simulink model "TD1_2"  (R2022b)
settings: Solver=VariableStepAuto  StartTime=0.0  StopTime=10.0  RelTol=1e-3
values from neighbouring files (symbols this model uses):
  A = [0 1; 1 2]    [temp.m]
  B = [0 ; 1]    [temp.m]
  C = [1 0]    [temp.m]
undefined symbols (not defined in the file or in its folder): h, K, Ki
settings Model: Creator=simon.dumesny  LastModifiedBy=simon.dumesny

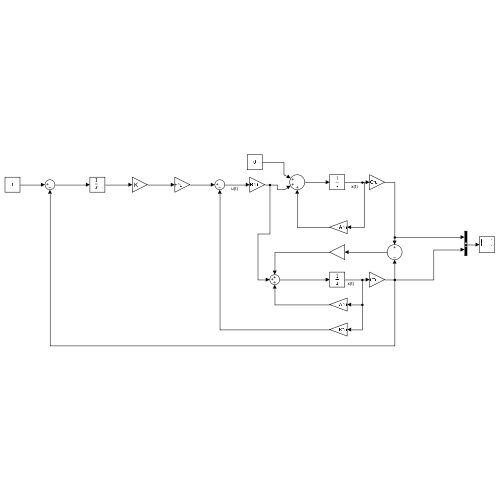
[thumbnail: Simulink's stored preview of the top-level diagram]
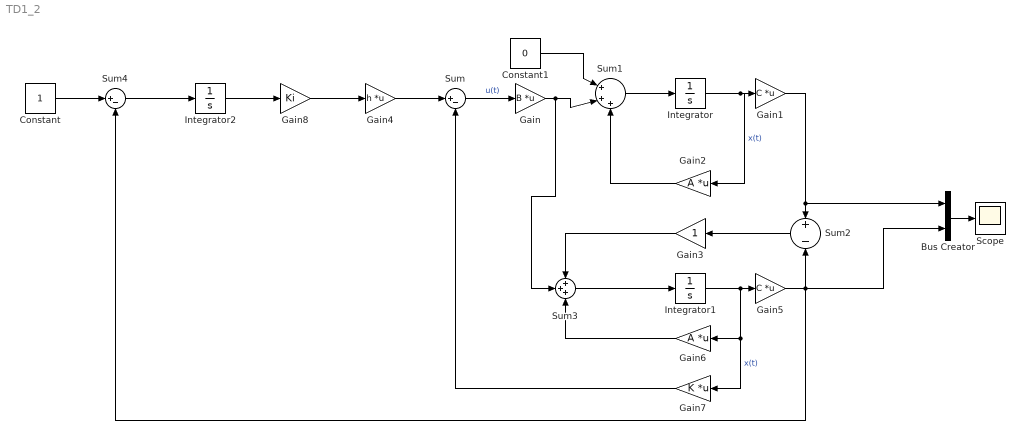
== system TD1_2 ==
  Bus Creator : BusCreator  Inputs=2
  Constant : Constant
  Constant1 : Constant  Value=0
  Gain : Gain  Gain=B  Multiplication=Matrix(K*u)
  Gain1 : Gain  Gain=C  Multiplication=Matrix(K*u)
  Gain2 : Gain  Gain=A  Multiplication=Matrix(K*u)
  Gain3 : Gain
  Gain4 : Gain  Gain=h  Multiplication=Matrix(K*u)
  Gain5 : Gain  Gain=C  Multiplication=Matrix(K*u)
  Gain6 : Gain  Gain=A  Multiplication=Matrix(K*u)
  Gain7 : Gain  Gain=K  Multiplication=Matrix(K*u)
  Gain8 : Gain  Gain=Ki
  Integrator : Integrator
  Integrator1 : Integrator
  Integrator2 : Integrator
  Scope : Scope
  Sum : Sum  Inputs=|+-
  Sum1 : Sum  Inputs=|+++
  Sum2 : Sum  Inputs=+-
  Sum3 : Sum  Inputs=+++
  Sum4 : Sum  Inputs=|+-
  wires:
  Sum/1 -> Gain/1  "u(t)"
  Gain/1 -> Sum3/2, Sum1/2
  Sum1/1 -> Integrator/1
  Constant1/1 -> Sum1/1
  Integrator/1 -> Gain2/1, Gain1/1  "x(t)"
  Gain2/1 -> Sum1/3
  Gain8/1 -> Gain4/1
  Gain4/1 -> Sum/1
  Gain1/1 -> Sum2/1, Bus Creator/1
  Bus Creator/1 -> Scope/1
  Sum2/1 -> Gain3/1
  Gain3/1 -> Sum3/1
  Sum3/1 -> Integrator1/1
  Integrator1/1 -> Gain7/1, Gain6/1, Gain5/1  "x(t)"
  Gain5/1 -> Sum2/2, Sum4/2, Bus Creator/2
  Gain6/1 -> Sum3/3
  Gain7/1 -> Sum/2
  Integrator2/1 -> Gain8/1
  Sum4/1 -> Integrator2/1
  Constant/1 -> Sum4/1
